simulink subsystem "fbw_law_blending"  (R2020b)
settings: Solver=VariableStepAuto  StartTime=0.0  StopTime=10.0  RelTol=1e-3
settings Model: Creator=Andreas  LastModifiedBy=Andreas

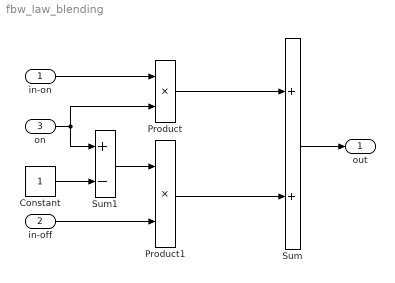
== system fbw_law_blending ==
  in-on : Inport
  in-off : Inport  Port=2
  on : Inport  Port=3
  Constant : Constant
  Product : Product
  Product1 : Product
  Sum : Sum
  Sum1 : Sum  Inputs=+-
  out : Outport
  wires:
  Product/1 -> Sum/1
  Product1/1 -> Sum/2
  Sum1/1 -> Product1/1
  in-on/1 -> Product/1
  in-off/1 -> Product1/2
  Sum/1 -> out/1
  on/1 -> Product/2, Sum1/1
  Constant/1 -> Sum1/2
